simulink model "ADRC_TWO_Order"  (Simulink 7.6)
settings: Solver=ode45  StartTime=0.0  StopTime=100  RelTol=1e-3
settings Model: Creator=Administrator  LastModifiedBy=Administrator
settings DebuggingCC: AlgebraicLoopMsg=none  ArtificialAlgebraicLoopMsg=none  SolverPrmCheckMsg=none  UnknownTsInhSupMsg=none

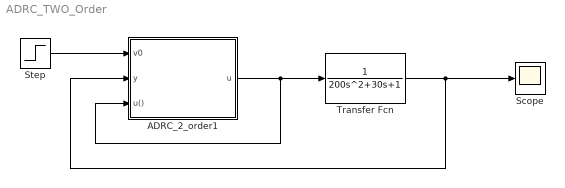
== system ADRC_TWO_Order ==
  ADRC_2_order1 : Subsystem  AncestorBlock=ADRC/ADRC/ADRC_2rd/ADRC_2_order1  mask{r0=0, h=0.01, B01=100, B02=300, B03=1000, D=0.01, b0=1, c=0.3, r1=5, h1=0.03}
      mask prompts: r0 "TD r0"; h "TD h"; B01 "B01="; B02 "B02="; B03 "B03="; D "D="; b0 "b0="; c "c="; r1 "r1="; h1 "h1="
  Scope : Scope
      settings: YMin=-200000  YMax=300000
  Step : Step  Time=0  SampleTime=0
  Transfer Fcn : TransferFcn  Denominator="[200  30 1]"
  wires:
  Step/1 -> ADRC_2_order1/1(v0)
  ADRC_2_order1/1(u) -> Transfer Fcn/1, ADRC_2_order1/3(u())
  Transfer Fcn/1 -> Scope/1, ADRC_2_order1/2(y)

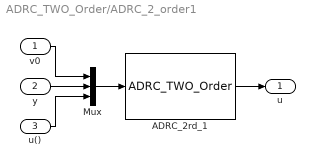
== system ADRC_TWO_Order/ADRC_2_order1 ==
  v0 : Inport
  y : Inport  Port=2
  u() : Inport  Port=3
  ADRC_2rd_1 : S-Function  FunctionName=ADRC_TWO_Order  Parameters=r0,h,B01,B02,B03,D,b0,c,r1,h1  EnableBusSupport=off
  Mux : Mux  Inputs=3
  u : Outport
  wires:
  ADRC_2rd_1/1 -> u/1
  v0/1 -> Mux/1
  y/1 -> Mux/2
  Mux/1 -> ADRC_2rd_1/1
  u()/1 -> Mux/3
